simulink model "PMRAC_time_delay_final"  (R2022a)
settings: Solver=VariableStepAuto  StartTime=0.0  StopTime=100  FixedStep=0.1  RelTol=1e-1  EnableMultiTasking=on
settings Model: Creator=Administrator  LastModifiedBy=mluser
settings SolverCC: AlgebraicLoopSolver=TrustRegion
settings DataIOCC: LimitDataPoints=on  SaveFormat=Array  ReturnWorkspaceOutputs=off
settings OptimizationCC: LifeSpan=inf
settings DebuggingCC: AlgebraicLoopMsg=none  SolverPrmCheckMsg=warning  UnconnectedInputMsg=warning  UnconnectedOutputMsg=warning  UnconnectedLineMsg=warning  AllowSymbolicDim=off  SFUnexpectedBacktrackingDiag=warning  SFNoUnconditionalDefaultTransitionDiag=warning  SFExecutionAtInitializationDiag=none  SFMachineParentedDataDiag=warning  ArithmeticOperatorsInVariantConditions=warning
settings HardwareCC: ProdBitPerPointer=32  ProdBitPerSizeT=32  ProdBitPerPtrDiffT=32  ProdLargestAtomicFloat=None  ProdIntDivRoundTo=Undefined  ProdEndianess=Unspecified  ProdWordSize=32  ProdHWDeviceType=32-bit Generic
settings ModelReferenceCC: PropagateSignalLabelsOutOfModel=off
settings SFSimCC: SimUseLocalCustomCode=off  CustomCodeUndefinedFunction=UseInterfaceOnly
settings RTWCC: RTWUseLocalCustomCode=off
settings CodeAppCC: StateflowObjectComments=on
settings GRTTargetCC: TargetLangStandard=C89/C90 (ANSI)
settings ConfigComp: CovMetricSettings=dw  CovSaveCumulativeToWorkspaceVar=on  CovSaveSingleToWorkspaceVar=on  CovExternalEMLEnable=off  CovSFcnEnable=off

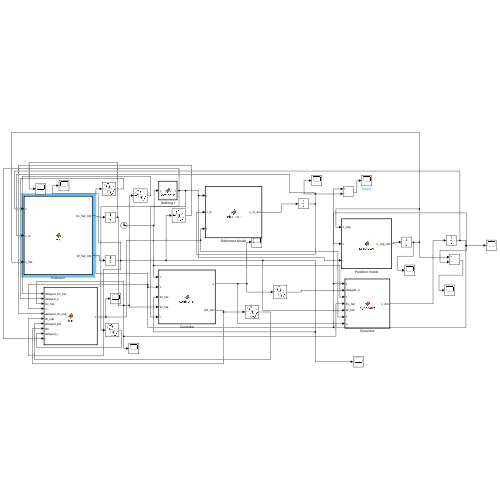
[thumbnail: Simulink's stored preview of the top-level diagram]
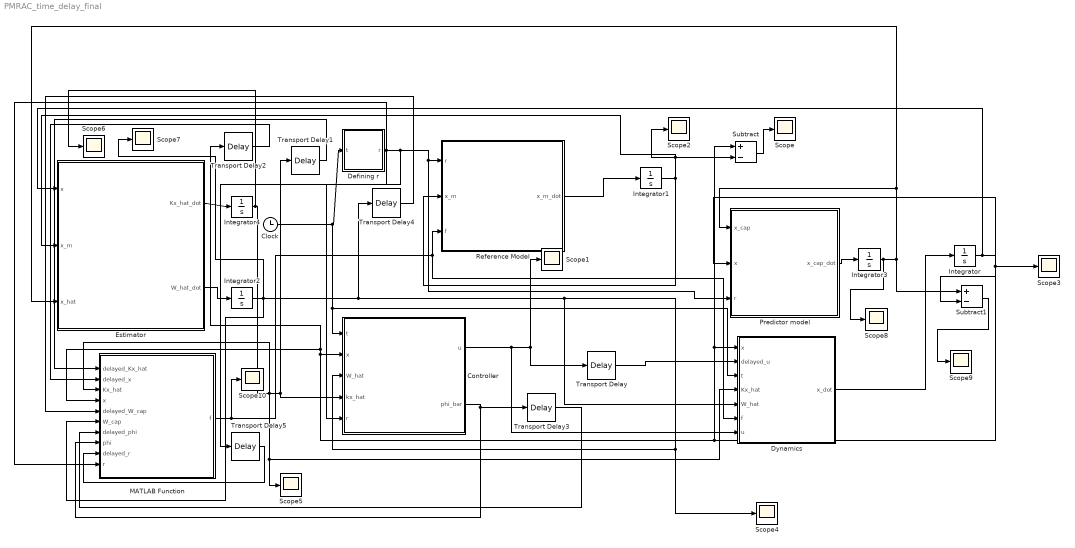
== system PMRAC_time_delay_final ==
  Clock : Clock
      settings: Decimation=50
  Controller : MATLAB Function  TreatAsAtomicUnit=on
  Defining r : MATLAB Function  TreatAsAtomicUnit=on
  Dynamics : MATLAB Function  TreatAsAtomicUnit=on
  Estimator : MATLAB Function  TreatAsAtomicUnit=on
  Integrator : Integrator  InitialCondition=[-1;1]
  Integrator1 : Integrator  InitialCondition=[0;0]
  Integrator2 : Integrator  InitialCondition=zeros(6,1)
  Integrator3 : Integrator  InitialCondition=[-1;1]
  Integrator4 : Integrator  InitialCondition=zeros(2,1)
  MATLAB Function : MATLAB Function  TreatAsAtomicUnit=on
  Predictor model : MATLAB Function  TreatAsAtomicUnit=on
  Reference Model : MATLAB Function  TreatAsAtomicUnit=on
  Scope{,1..10} (11 alike) : Scope
  Subtract : Sum  Inputs=+-
  Subtract1 : Sum  Inputs=+-
  Transport Delay{,1..5} (6 alike) : TransportDelay  DelayTime=0
  wires:
  Dynamics/1(x_dot) -> Integrator/1
  Integrator/1 -> Estimator/1(x), Subtract1/2, Scope3/1, Predictor model/2(x), Subtract/1, Dynamics/1(x), MATLAB Function/4(x), Transport Delay2/1, Controller/2(x)
  Clock/1 -> Defining r/1(t), Dynamics/3(t), Controller/1(t)
  Controller/1(u) -> Dynamics/7(u), Transport Delay/1, Scope1/1
  Reference Model/1(x_m_dot) -> Integrator1/1
  Integrator1/1 -> Estimator/2(x_m), Subtract/2, Scope2/1, Reference Model/2(x_m)
  Integrator2/1 -> Scope7/1, Scope4/1, Controller/3(W_hat), Dynamics/5(W_hat), Transport Delay4/1, MATLAB Function/6(W_cap)
  Subtract/1 -> Scope/1
  Predictor model/1(x_cap_dot) -> Integrator3/1
  Integrator3/1 -> Scope8/1, Subtract1/1, Estimator/3(x_hat), Predictor model/1(x_cap)
  Estimator/2(W_hat_dot) -> Integrator2/1
  Estimator/1(Kx_hat_dot) -> Integrator4/1
  Integrator4/1 -> Scope6/1, Scope5/1, Dynamics/4(Kx_hat), MATLAB Function/3(Kx_hat), Transport Delay1/1, Controller/4(kx_hat)
  Transport Delay/1 -> Dynamics/2(delayed_u)
  MATLAB Function/1(f) -> Scope10/1, Reference Model/3(f), Dynamics/6(f)
  Transport Delay1/1 -> MATLAB Function/1(delayed_Kx_hat)
  Transport Delay2/1 -> MATLAB Function/2(delayed_x)
  Transport Delay4/1 -> MATLAB Function/5(delayed_W_cap)
  Controller/2(phi_bar) -> Transport Delay3/1, MATLAB Function/8(phi)
  Transport Delay3/1 -> MATLAB Function/7(delayed_phi)
  Transport Delay5/1 -> MATLAB Function/9(delayed_r)
  Defining r/1(r) -> MATLAB Function/10(r), Controller/5(r), Predictor model/3(r), Reference Model/1(r), Transport Delay5/1
  Subtract1/1 -> Scope9/1

== matlab function PMRAC_time_delay_final/Defining r ==
  data: t input; r output
function r   = define_r(t)
r = sin(t);

== matlab function PMRAC_time_delay_final/Controller ==
  data: u output; t input; x input; W_hat input; kx_hat input; r input; phi_bar output
function [u,phi_bar]   = controller(t,x,W_hat,kx_hat,r)

%r=10;
%r=exp(-t);

%r=sin(t);

%k_x=[-2/3 -1/3]'; % note that the linear control gain is directly chosen instead of adapting with an assumption of $A$ matrix to be known
theta=x(1,1);
p=x(2,1);
phi_bar = [1; theta; p; abs(theta)*p; abs(p)*p; theta^3];

u=kx_hat'*x-W_hat'*phi_bar+r;

end

== matlab function PMRAC_time_delay_final/Dynamics ==
  data: x input; delayed_u input; x_dot output; t input; Kx_hat input; W_hat input; f input; u input
function x_dot = dynamics(x,delayed_u,t,Kx_hat,W_hat,f,u)

L_delta_a=1;

A=[0 1; 0 0];

a0=0.8;
a1=0.2314;
a2=0.6918;
a3=-0.6245;
a4=0.0095;
a5=0.0214;

B=[0 1]';

theta=x(1,1);
p=x(2,1);

W = [a0;a1;a2;a3;a4;a5];
phi_bar = [1; theta; p; abs(theta)*p; abs(p)*p; theta^3];
%phi_bar =[1;1;1;1;1;1];

A_ref = [0,1;-2,-1];
%Bc = [0;1];
%r = sin(t);
lambda = 1;
Kx = [2;6];
delta=a0+a1*theta+a2*p+a3*abs(theta)*p+a4*abs(p)*p+a5*theta^3;
%x_dot=A*x+B*lambda*(delayed_u+W'*phi_bar);
%x_dot = A_ref*x+B*lambda*(Kx_hat'*x-Kx'*x-W_hat'*phi_bar+W'*phi_bar)+f;
x_dot = A*x + B*(u+delta/L_delta_a);
end

== matlab function PMRAC_time_delay_final/Predictor model ==
  data: x_cap_dot output; x_cap input; x input; r input
function x_cap_dot = predictor( x_cap, x, r)


am1=-2;
am2=-1;
A_ref=[0 1; am1 am2];

A_prd =4* A_ref;


L_delta_a=1;
B_c=[0; L_delta_a];

x_cap_dot = A_prd*(x_cap-x) + A_ref*x + B_c*r;

== matlab function PMRAC_time_delay_final/Reference Model ==
  data: r input; x_m_dot output; x_m input; f input
function x_m_dot   = reference(r,x_m,f)
am1=-2;
am2=-1;
L_delta_a=1;
%r=exp(-t);
%r=sin(t);
%r=2*sin(t);
%A_ref=A+B*k_x';
A_ref=[0 1; am1 am2];
B_c=[0; L_delta_a];
x_m_dot=A_ref*x_m+f+B_c*r;

== matlab function PMRAC_time_delay_final/MATLAB Function ==
  data: delayed_Kx_hat input; f output; delayed_x input; Kx_hat input; x input; delayed_W_cap input; W_cap input; delayed_phi input; phi input; delayed_r input; r input
function f = fcn(delayed_Kx_hat,delayed_x,Kx_hat,x,delayed_W_cap,W_cap,delayed_phi,phi,delayed_r,r)
B = [0;1];
lambda = 1;

f = B*lambda*(delayed_Kx_hat'*delayed_x-Kx_hat'*x-delayed_W_cap'*delayed_phi+W_cap'*phi+delayed_r-r);

== matlab function PMRAC_time_delay_final/Estimator ==
  data: Kx_hat_dot output; W_hat_dot output; x input; x_m input; x_hat input
function [Kx_hat_dot, W_hat_dot] = fcn(x, x_m, x_hat)

%gamma_x = [1,0;
 %          2,1];
gamma_x=2*eye(2);
%gamma_w = [1,0,1,2,3,4;
  %         3,4,1,2,5,6;
  %         5,2,1,6,8,3;
  %         2,4,5,7,2,1;
  %         4,5,1,2,6,3;
  %         7,9,0,1,3,0];
gamma_w=10*eye(6);

theta=x(1,1);
p=x(2,1);
phi_bar = [1; theta; p; abs(theta)*p; abs(p)*p; theta^3];

%P_ref = [1.75,-0.5;-0.5,3];s
%P_ref=[3.5 0.5;0.5 1.5];
P_ref = [8.75,1.25;1.25,3.75];

P_prd =4* P_ref;
B=[0 1]';


Kx_hat_dot = -gamma_x*x*((x-x_m)'*P_ref-(x_hat-x)'*P_prd)*B;
W_hat_dot = gamma_w*phi_bar*((x-x_m)'*P_ref-(x_hat-x)'*P_prd)*B;

%Kx_hat_dot = -gamma_x*x*((x-x_m)'*P_ref)*B;
%W_hat_dot = gamma_w*phi_bar*((x-x_m)'*P_ref)*B;
